simulink model "CML_DynamicProprioTest"  (R2015a)
settings: Solver=ode4  SolverMode=MultiTasking  StartTime=0.0  StopTime=inf  FixedStep=BKIN_STEP_TIME  RelTol=1e-3
StartFcn:
  |  warndlg('Dexterit-E models cannot run under simulation. Please compile your model and run it from within Dexterit-E.');set_param(bdroot,'SimulationCommand','stop')
model workspace (MAT data in the model file):
  col_x = 1
  col_y = 2
  RADIUS_VIS = 3
  COLOR_INIT = 4
  BKIN_STEP_TIME = 0.00025
  START_WAIT_TIME_COL = 3
  E_END_TRIAL = 20
  STROKE_WIDTH = 6
  K_HAND_VEL = 1
  K_HOLDTIME = 2
  K_ROBOT_RAMP_TIME = 3
  E_ENABLED_CONTROLLER = 31
  K_TIME_TO_START = 4
  BKIN_KINEMATIC_FRAME_SIZE = 400
  E_NO_EVENT = 0
  ROTATION = 7
  E_WAIT_JS_THRESH = 16
  E_AT_JS_THRESH = 18
  STARTTARGET_COL = 1
  TIME_RETURNTOSTART_COL = 2
  MOVE_TIME_COL = 4
  TARGET_SHIFTTIME_COL = 5
  SHOWTARGETDUR_COL = 7
  MOVE_XVEL_COL = 9
  MOVE_YVEL_COL = 10
  E_INIT_TRIAL = 1
  E_MOVE_TO_START = 2
  E_AT_START = 4
  E_PASSIVE_HOLD_AT_START = 6
  E_MOVE_TO_END = 8
  COLOR_SELECT = 5
  ACTORPAS_COL = 11
  E_AT_END = 10
  DELAY_POSTTRIAL_COL = 8
  TARGETSHIFTDIR_COL = 6
  LABEL_HEIGHT = 8
  LABEL = 9
  E_ACTIVE_HOLD_AT_START = 7
  MVMT_VTHRESH_LB = 12
  MVMT_VTHRESH_UB = 13
  CHANNEL_WIDTH = 1
  WALL_WIDTH = 2
  WALL_STIFFNESS = 3
  WALL_VISCOSITY = 4
  E_STOP_MOVING = 21
undefined symbols (not defined in the file): slselsubs
libraries: Video x6, simulink x5, slrtlib x5, General x3, KINARM_loads x3, KINARM_general x2, KINARM_IO x1, xpcnilib x1
(part 2 of 2)

== stateflow chart CML_DynamicProprioTest/Trial Control ==
  state Main/
    state InitTrial/
      event_code=E_INIT_TRIAL;
      StartPos[1] = CurHandPos[1];
      StartPos[2] = CurHandPos[2];
      EndPos[1] = Target_Table[Trial_Protocol[STARTTARGET_COL]][1];
      EndPos[2] = Target_Table[Trial_Protocol[STARTTARGET_COL]][2];
      MoveTime = Trial_Protocol[TIME_RETURNTOSTART_COL];
      HandWindowState = 0;
      //enable_controller = 0;
      t_step = 0;
      tone = 0;
      logging_enable = 0;
    state MoveArmToStartTarget/
      event_code=E_MOVE_TO_START;
      enable_controller = 1;
      trajtype = 0;  //set to 1 to be constant velocity, set to 0 to be bezier
      ForceChannelState = 0; //turn off the force channel
      ForceScale = 1; //let the automatic ramp take care of turning the forces on
      t_step = 0;
      //increment t_step on each clock cycle
      during:
      on e_clk: t_step = t_step + (1/ (MoveTime/1000 * 1000));
    state HoldAtStart/
      event_code=E_AT_START;
      ShowHand = 1;
      tickCount = 500;
      TextState = 0;
      //reset all the move and shift parameters
      StartTarget = Trial_Protocol[STARTTARGET_COL];
      StartPos[1] = Target_Table[StartTarget][1];
      StartPos[2] = Target_Table[StartTarget][2];
      MoveVel[1] = 0;
      MoveVel[2] = 0;
      MoveTime = 0;
      TargetShiftTime = 0;
      ShowTime =0;
      direction = 0;
      HandPosShift[1] = 0;
      HandPosShift[2] = 0;
      logging_enable = 1;
    state SelectActorPas/
      AorP = Trial_Protocol[ACTORPAS_COL];
    state ActiveHoldAtStart/
      event_code=E_ACTIVE_HOLD_AT_START;
      enable_controller = 0;
      ForceScale = 0;
      t_step = 0;
      HandWindowState = 1;
      ShowHand = 1;
      trajtype = 1;
      tickCount = Trial_Protocol[START_WAIT_TIME_COL];
    state HandOutOfWindow/
      //wait until hand is back in the window
    state PassiveHoldAtStart1/
      event_code=E_PASSIVE_HOLD_AT_START;
      enable_controller = 1;
      t_step = 0;
      trajtype = 1;  //set to 1 to be constant velocity, set to 0 to be bezier
      tickCount = Trial_Protocol[START_WAIT_TIME_COL];
    state ActiveStart/
      event_code=E_AT_START;
      ShowHand = 1;
      tickCount = 200;
    state PassiveHoldNoTarget/
      ShowHand = 0;
      tickCount = 200;
      //set up the target shift parameters
      MoveVel[1] = Trial_Protocol[MOVE_XVEL_COL];
      MoveVel[2] = Trial_Protocol[MOVE_YVEL_COL];
      MoveTime = Trial_Protocol[MOVE_TIME_COL];
      TargetShiftTime = Trial_Protocol[TARGET_SHIFTTIME_COL];
      direction = Trial_Protocol[TARGETSHIFTDIR_COL];
      ShowTime = Trial_Protocol[SHOWTARGETDUR_COL];
      TShowStart = 0.5-((ShowTime/2)/MoveTime);
      TShowEnd = 0.5+((ShowTime/2)/MoveTime);
      //the X shift is Vx*tshift*cos(dir) + Vy*tshift*sin(dir), and similarly for the Y shift
      //the direction should be relative to the direction of motion defined by Vx,Vy
      movdir = atan2(MoveVel[2],MoveVel[1]) * 180/pi;
      direction = direction; //+ movdir;
      HandPosShift[1] = (TargetShiftTime/1000)*MoveVel[1]*cos(direction*pi/180) + -(TargetShiftTime/1000)*MoveVel[2]*sin(direction*pi/180);
      HandPosShift[2] = (TargetShiftTime/1000)*MoveVel[1]*sin(direction*pi/180) + (TargetShiftTime/1000)*MoveVel[2]*cos(direction*pi/180);
      trajtype = 1;  //set to 1 to be constant velocity, set to 0 to be bezier
      t_step = 0;
      exit:
      tone = 1;
    state GoCue/
      ShowHand = 0;
      HandWindowState = 0;
      tone = 1;
      tickCount = 0;
      //set up the target shift parameters
      MoveVel[1] = Trial_Protocol[MOVE_XVEL_COL];
      MoveVel[2] = Trial_Protocol[MOVE_YVEL_COL];
      MoveTime = Trial_Protocol[MOVE_TIME_COL];
      TargetShiftTime = Trial_Protocol[TARGET_SHIFTTIME_COL];
      direction = Trial_Protocol[TARGETSHIFTDIR_COL];
      ShowTime = Trial_Protocol[SHOWTARGETDUR_COL];
      EndPos[1] = Target_Table[StartTarget][1] + (MoveVel[1]*100)*(MoveTime/1000*2); // (m/s to cm/s), multiply by (ms to s) to get cm
      EndPos[2] = Target_Table[StartTarget][2] + (MoveVel[2]*100)*(MoveTime/1000*2); // (m/s to cm/s), multiply by (ms to s) to get cm
      TShowStart = MoveTime/2 - (ShowTime/2);
      TShowEnd = MoveTime/2 + (ShowTime/2);
      //the X shift is Vx*tshift*cos(dir) + Vy*tshift*sin(dir), and similarly for the Y shift
      //the direction should be relative to the direction of motion defined by Vx,Vy
      movdir = atan2(MoveVel[2],MoveVel[1]) * 180/pi;
      direction = direction; //+ movdir;
      //here we will use the ideal movement velocity rather than the true movement velocity so that the shift is constant during the trial...
      HandPosShift[1] = (TargetShiftTime/1000)*MoveVel[1]*cos(direction*pi/180) + -(TargetShiftTime/1000)*MoveVel[2]*sin(direction*pi/180);
      HandPosShift[2] = (TargetShiftTime/1000)*MoveVel[1]*sin(direction*pi/180) + (TargetShiftTime/1000)*MoveVel[2]*cos(direction*pi/180);
      trajtype = 0;  //set to 1 to be constant velocity, set to 0 to be bezier
      //turn on the force channel
      ForceChannelState = 1; //turn on the force channel
    state MoveArm/
      event_code=E_MOVE_TO_END;
      during:
      on e_clk: t_step = t_step + (1/ (MoveTime/1000 * 1000));
      ShowHand = ((t_step > TShowStart) && (t_step <= TShowEnd));
    state DuringActiveMovement/
      event_code=E_MOVE_TO_END;
      vthreshMax = 0;
      vthreshMin = 0;
      tickCount = 0;
      vthreshUB = sqrt(MoveVel[1]^2 + MoveVel[2]^2) + sqrt(MoveVel[1]^2 + MoveVel[2]^2)*.2; //Trial_Protocol[MVMT_VTHRESH_UB];
      vthreshLB = sqrt(MoveVel[1]^2 + MoveVel[2]^2) - sqrt(MoveVel[1]^2 + MoveVel[2]^2)*.2; //Trial_Protocol[MVMT_VTHRESH_LB];
      during:
      tickCount++;
      ShowHand = ((tickCount > TShowStart) && (tickCount <= TShowEnd));  //compute in real time
      HandVel = sqrt(HandVelocity[1]^2 + HandVelocity[2]^2);
      vthreshMax = vthreshMax || (HandVel > vthreshUB); //true if you ever exceed UB
      vthreshMin = vthreshMin || (HandVel > vthreshLB); //true if you ever exceed LB
    state HoldAtEnd/
      event_code=E_AT_END;
      t_step = 1;
      ShowHand = 0;
    state StopActiveMovement/
      event_code = E_STOP_MOVING;
      //if we have moved long enough, catch the hand to stop it from moving
      enable_controller = 1;  //turn on the position controller to catch the hand
      ForceChannelState = 0; //turn off the force channel
      trajtype = 0;  //set to 1 to be constant velocity, set to 0 to be bezier
      StartPos[1] = CurHandPos[1]; //+HandVelocity[1]*100*.2;
      StartPos[2] = CurHandPos[2]; //+HandVelocity[2]*100*.2;
      ShowHand = 0;
      during:
      ForceScale = ForceScale + 0.002;
      //StartPos[1] = CurHandPos[1];
      //StartPos[2] = CurHandPos[2];
    state TimeAtThresh/
      event_code = E_AT_JS_THRESH;
      tickCount = 300;
    state WaitForThreshold/
      event_code = E_WAIT_JS_THRESH;
      visAid_State[1] =1; visAid_State[2] =0;
      visAid_State[3] =1; visAid_State[4] =0;
      response = joystick;
      during:
      response = joystick;
    state TooFast/
      TextState = 2;
    state JustRight/
      TextState = 0;
    state TooSlow/
      TextState = 1;
    state EndOfTrial/
      event_code = E_END_TRIAL;
      StartPos[1] = CurHandPos[1];
      StartPos[2] = CurHandPos[2];
      trajtype = 0;  //set to 1 to be constant velocity, set to 0 to be bezier
      t_step = 0;
      tickCount =Trial_Protocol[DELAY_POSTTRIAL_COL];
      tone = 0;
    InitTrial -> MoveArmToStartTarget : after(200,e_clk)
    MoveArmToStartTarget -> HoldAtStart : // t done incrementing
        | [(t_step >= 1)]/
        | t_step = 1;
    HoldAtStart -> SelectActorPas : after(tickCount, e_clk)
    SelectActorPas -> PassiveHoldAtStart1 [order 1] : //passive condition
        | [AorP <= 0]
    SelectActorPas -> ActiveHoldAtStart [order 2] : //active condition
        | [AorP > 0]
    HandOutOfWindow -> ActiveHoldAtStart : [HandInTarget[StartTarget] == 1]
    ActiveHoldAtStart -> HandOutOfWindow [order 1] : [HandInTarget[StartTarget] == 0]
    ActiveHoldAtStart -> ActiveStart [order 2] : after(tickCount, e_clk)
    PassiveHoldAtStart1 -> PassiveHoldNoTarget : after(tickCount, e_clk)
    ActiveStart -> GoCue : after(tickCount,e_clk)
    PassiveHoldNoTarget -> MoveArm : after(tickCount,e_clk)
    GoCue -> DuringActiveMovement : [HandInTarget[StartTarget] == 0]
    MoveArm -> HoldAtEnd : // t done incrementing
        | [(t_step >= 1)]/
        | t_step = 1;
    DuringActiveMovement -> StopActiveMovement : [tickCount > MoveTime]
    HoldAtEnd -> WaitForThreshold : after(50,e_clk)
    StopActiveMovement -> (junction 675) : [ForceScale >= 1]/
        | ForceScale = 1;
        | event_code=E_AT_END;
    (junction 675) -> TooFast [order 2] : [vthreshMax > 0]
    (junction 675) -> TooSlow [order 1] : [vthreshMin == 0]
    (junction 675) -> JustRight [order 3] : [vthreshMin > 0 && vthreshMax == 0]
    WaitForThreshold -> TimeAtThresh : [after(1,e_clk) && (response == 1 || response == 3)]/
        | visAid_State[response] = 2;
        | //only happens if past thresh
    TimeAtThresh -> WaitForThreshold [order 2] : [after(1,e_clk) && (joystick < 1  || response ~= joystick)]/
        | visAid_State[response] = 1;
        | response = 0;
    (junction 678) -> WaitForThreshold : after(50,e_clk)
    TooFast -> (junction 678)
    JustRight -> (junction 678)
    TooSlow -> (junction 678)
    TimeAtThresh -> EndOfTrial [order 1] : [after(tickCount,e_clk)]/
        | visAid_State[1] =0; visAid_State[2] =0;
        | visAid_State[3] =0; visAid_State[4] =0;
  state init/
    ramp_time = TaskwideParams[K_ROBOT_RAMP_TIME];
    enable_controller = 0;
    tone = 0;
    response = 0;
    visAid_State[1] = 0;visAid_State[2] = 0;visAid_State[3] = 0;visAid_State[4] = 0;
    EndPos[1] = 0;
    EndPos[2] = 0;
    ForceScale = 0;
    TextState = 0;
    ForceChannelState = 0; //turn off the force channel
    trajtype = 0;  //set to 1 to be constant velocity, set to 0 to be bezier
    logging_enable = 0;
  state Inter_Trial_State1/
    //reset the event code, and send the
    //e_Trial_End Stateflow event to indicate that the trial is over.
    event_code = 0;
    tickCount = 100;
    e_Trial_End;
  state RobotRampDown/
    enable_controller = 0;
    ramp_time = 2000;
  (default) -> init
  init -> InitTrial
  Inter_Trial_State1 -> InitTrial : // has a a specified period of
      | // time occured?
      | after(tickCount, e_clk)
  Main -> RobotRampDown : e_ExitTrialNow/
      | tickCount = 1;
      | // e_ExitTrialNow event occurs if the
      | // Dex pause is pressed by the operator
  RobotRampDown -> Inter_Trial_State1 : after(ramp_time,e_clk)
  EndOfTrial -> Inter_Trial_State1 : after(100, e_clk)
  data: logging_enable output double; event_code output uint16 [0..] =0; AorP output double; enable_controller output double; ForceScale output double [0..1]; direction output double; tickCount local double; Trial_Protocol input double; HandInTarget input double; TaskwideParams input double; HandVelocity input double; t_step output double size=1; StartPos output double size=[1 2]; MoveVel output double size=[1 2]; EndPos output double size=[1 2]; trajtype output double size=1; ForceChannelState output double; ShowHand output double size=1; HandPosShift output double size=[1 2]; movdir output double; StartTarget output double; HandWindowState output double; TextState output double; visAid_State output double size=[1 4]; Target_Table input double size=[64 25]; CurHandPos input double size=[1 2]; joystick input int32 size=1; response output double size=1; TShowStart output double; TShowEnd output double; tone output double size=1; Repeat_Trial_Flag output boolean; MoveTime local double; ShowTime local double; TargetShiftTime local double; pi parameter double =3.141592653589793; vthreshMax local double; vthreshMin local double; ramp_time local double; HandVel local double; vthreshUB local double; vthreshLB local double
  events: e_clk input RISING_EDGE_EVENT; e_ExitTrialNow input EITHER_EDGE_EVENT; e_Trial_End output EITHER_EDGE_EVENT

== matlab function CML_DynamicProprioTest/MakeTraj/pos_velramp ==
  data: startxy input size=[1 2]; handvel input; t input; desiredPos output size=[1 2]; VCODE input; VCODE_mod output
function [desiredPos,VCODE_mod] = fcn(startxy,handvel,t,VCODE)
%#codegen

%xy position in cm, velocity in m/s

startxy = startxy/100; %convert to meters

xvel = handvel(1);
yvel = handvel(2);

VCODE_mod = VCODE;

%clip t just in case!
if t < 0
    t = 0;
elseif t > 1;
    t = 1;
end

%we will spend the first 10% of the movement accelerating and the last 10%
%of the movement decelerating. we will use a trapezoidal profile for
%simplicity

xshift = 0;
yshift = 0;

if t < 0.1
    
    %xshift = 0.5*xvel*t;
    %yshift = 0.5*yvel*t;
    xshift = xvel/(.2)*t^2;
    yshift = yvel/(.2)*t^2;
    
elseif t < 0.9

    %xshift = 0.5*xvel*0.1 + (t-0.1)*xvel;
    %yshift = 0.5*yvel*0.1 + (t-0.1)*yvel;
    xshift = xvel/(.2)*0.1^2 + (t-0.1)*xvel;
    yshift = yvel/(.2)*0.1^2 + (t-0.1)*yvel;
    
elseif t <= 1

    %xshift = 0.5*xvel*0.1 + (t-0.1)*xvel + 0.5*xvel*(t-0.9);
    %yshift = 0.5*yvel*0.1 + (t-0.1)*yvel + 0.5*yvel*(t-0.9);
    xshift = xvel/(.2)*0.1^2 + (t-0.1)*xvel + xvel/(0.2)*(t-0.9)^2;
    yshift = yvel/(.2)*0.1^2 + (t-0.1)*yvel + yvel/(0.2)*(t-0.9)^2;
    
end

xpos = startxy(1)+xshift;
ypos = startxy(2)+yshift;

desiredPos = [xpos ypos];

VCODE_mod(1,3) = desiredPos(1); %convert to meters
VCODE_mod(1,4) = desiredPos(2); %convert to meters

== stateflow chart CML_DynamicProprioTest/Subsystem2/Chart ==
  state EnableState/
    state AutoMoveToPos/
      //smoothly creates a trajectory to get the hand to a point eventually
      state MovingToDesiredXY/
        tickCount = TaskwideParams[K_TIME_TO_START];
        state = 11;
        tick = 0;
        during:
        on e_clk: tick++;
        // the trajectory velocity will have a bell shaped profile
        trajectory_shape = tick/tickCount-sin(2*pi*tick/tickCount)/(2*pi);
        virtual_pos[1] = StartPos[1] + (TgtPos[1] - StartPos[1]) * trajectory_shape;
        virtual_pos[2] = StartPos[2] + (TgtPos[2] - StartPos[2]) * trajectory_shape;
      state GetDesiredXY/
        //grab the current desired pos in case it changes
        TgtPos[1] = DesiredPos[1];
        TgtPos[2] = DesiredPos[2];
        StartPos[1] = HandPos[1];
        StartPos[2] = HandPos[2];
        updatepos = 0;
        state = 10;
      state HoldAtDesiredXY/
        //pause until something changes
        state = 12;
        updatepos = 0;
        during:
        on e_clk: updatepos = ( (abs(TgtPos[1]-DesiredPos[1]) > 0.01) || (abs(TgtPos[2]-DesiredPos[2]) > 0.01) )
      GetDesiredXY -> MovingToDesiredXY : after(1, e_clk)
      HoldAtDesiredXY -> GetDesiredXY : [updatepos == 1 && MovOnTraj == 0]
      MovingToDesiredXY -> HoldAtDesiredXY : after(tickCount, e_clk)/
    state MoveAlongTraj/
      //take a step along a trajectory specified externally
      state GetDesiredXY_Traj/
        TgtPos[1] = DesiredPos[1];
        TgtPos[2] = DesiredPos[2];
        StartPos[1] = HandPos[1];
        StartPos[2] = HandPos[2];
        state = 21;
        //movIsSafe = ( (abs(TgtPos[1]-HandPos[1]) < 0.02) || (abs(TgtPos[2]-HandPos[2]) < 0.02) );
        movIsSafe = 1;
      state MovAlongTraj/
        state = 22;
        virtual_pos[1] = DesiredPos[1];
        virtual_pos[2] = DesiredPos[2];
      GetDesiredXY_Traj -> MovAlongTraj [order 2] : [movIsSafe == 1]
      MovAlongTraj -> GetDesiredXY_Traj
    (junction 15) -> GetDesiredXY [order 1] : [MovOnTraj == 0]
    (junction 15) -> GetDesiredXY_Traj [order 2] : [MovOnTraj == 1]
    MoveAlongTraj -> GetDesiredXY : [MovOnTraj == 0]
    GetDesiredXY_Traj -> GetDesiredXY [order 1] : [movIsSafe == 0]
    AutoMoveToPos -> GetDesiredXY_Traj : [MovOnTraj == 1]
  state Init/
    ramp_time = TaskwideParams[K_ROBOT_RAMP_TIME];
    scale_increment = 1/ramp_time;
    force_scale = 0;
    state = 1;
    during:
    CurHandPos[1] = HandPos[1];
    CurHandPos[2] = HandPos[2];
  state RampUp/
    //ramp up the force scale to 1
    CurHandPos[1] = HandPos[1];
    CurHandPos[2] = HandPos[2];
    virtual_pos[1] = HandPos[1];
    virtual_pos[2] = HandPos[2];
    state = 2;
    force_scale = 0;
    during:
    on e_clk: force_scale += scale_increment;
  state ResetController/
    reset_controller;
  state RampDown/
    //ramp down the force scale to 1
    CurHandPos[1] = HandPos[1];
    CurHandPos[2] = HandPos[2];
    virtual_pos[1] = CurHandPos[1];
    virtual_pos[2] = CurHandPos[2];
    state = 30
    during:
    on e_clk: force_scale -= scale_increment;
  (default) -> Init
  Init -> ResetController : //if controller becomes enabled
      | [enable_controller == 1]/
      | force_scale = 0;
  ResetController -> RampUp
  RampUp -> (junction 15) [order 2] : [force_scale >= 1]/
      | force_scale = 1;
  RampDown -> Init [order 2] : [force_scale <0]/
      | force_scale = 0;
  RampDown -> RampUp [order 1] : [enable_controller == 1]
      | //if the controller is enabled
  RampUp -> RampDown [order 1] : [enable_controller == 0]
      | //if the controller gets shut off
  EnableState -> RampDown : [enable_controller == 0]
  data: enable_controller input double; DesiredPos input; HandPos input; TaskwideParams input; force_scale output double; virtual_pos output double size=2; tickCount local double; StartPos local double size=2; TgtPos local double size=2; updatepos local boolean; MovOnTraj input double; CurHandPos local double size=2; ramp_time local double; scale_increment local double; tick local double; trajectory_shape local double; movIsSafe local boolean; pi constant double =3.14159265358979; state output double
  events: e_clk input EITHER_EDGE_EVENT; reset_controller output EITHER_EDGE_EVENT

== matlab function CML_DynamicProprioTest/Subsystem2/MATLAB Function ==
  data: pos input; VCODE_MOD output; VCODE input
function VCODE_MOD = fcn(pos,VCODE)
%#codegen

VCODE_MOD = VCODE;

VCODE_MOD(3) = pos(1);
VCODE_MOD(4) = pos(2);

== matlab function CML_DynamicProprioTest/TextFeedback/MATLAB Function ==
  data: VCODE input; VCODE_MOD output; texttype input
function VCODE_MOD  = rwd_tgt(VCODE,texttype)
%#codegen

%give feedback (too fast/too slow)

VCODE_MOD = VCODE;

text = '';
if texttype == 1
    text = 'Too Slow!';
elseif texttype == 2
    text = 'Too Fast!';
end

textnum = double(text); %this quickly casts each char into a number

%make sure we won't overflow the VCODE: no more than 50 chars! we will
%clip off anything that overflows.
VCODE_MOD(1,15:min([15+length(text),64])) = textnum(1:min([length(textnum),50])); %write out as many the characters as possible into the VCODE
VCODE_MOD(1,min([15+length(text)+1,64])) = 0;  %terminate the string!

== matlab function CML_DynamicProprioTest/MakeTraj/PassThrough ==
  data: startxy input; pos output; VCODE input; VCODE_mod output
function [pos,VCODE_mod] = fcn(startxy,VCODE)
%#codegen

%this function passes the input directly to the output. 
%NOTE, THIS CAN BE VERY DANGEROUS TO ENGAGE, AS IT DOES NOT SHAPE THE
% OUTPUT "NICELY" BEFORE SENDING IT TO THE POSITION CONTROLLER 

VCODE_mod = VCODE;

pos = startxy/100;  %convert cm to m

VCODE_mod(1,3) = pos(1);
VCODE_mod(1,4) = pos(2);
